simulink model "testMPC"  (R2019a)
settings: Solver=VariableStepAuto  StartTime=0.0  StopTime=10000  RelTol=1e-3
values from neighbouring files (symbols this model uses):
  Afault1_2 = [-0.0777422601611 0 0.00516641602336 0 0 0 0 0 0 1 0 0.364315718282 ... (121 elements, 11x11)]    [UpdatedWorkspace.mat]    (also in current.mat; current2.mat; finalWorkspace.mat; genTestingData.m = [-0.0777422601610909,0.364315718281914,0,-49.5311012194985,0)
  Bfault1_2 = [0 -0.116933195054 -1.86328082403 0 0 0 0 0 0 0 0 0 ... (44 elements, 11x4)]    [UpdatedWorkspace.mat]    (also in current.mat; current2.mat; finalWorkspace.mat; genTestingData.m = [0,0,0,0)
  C = [1 0 0 0 0 0 0 0 0 0 0 ... (first row only)    [chanceConstraintProgramming4.m]    (also in current.mat = [1 0 0 0 0 0 0 0 0 0 0 0 ... (44 elements, 4x11)]; current2.mat = [1 0 0 0 0 0 0 0 0 0 0 0 ... (44 elements, 4x11)])
undefined symbols (not defined in the file or in its folder): testA, testB
libraries: mpclib x1
settings Model: Creator=mschr  LastModifiedBy=mschr

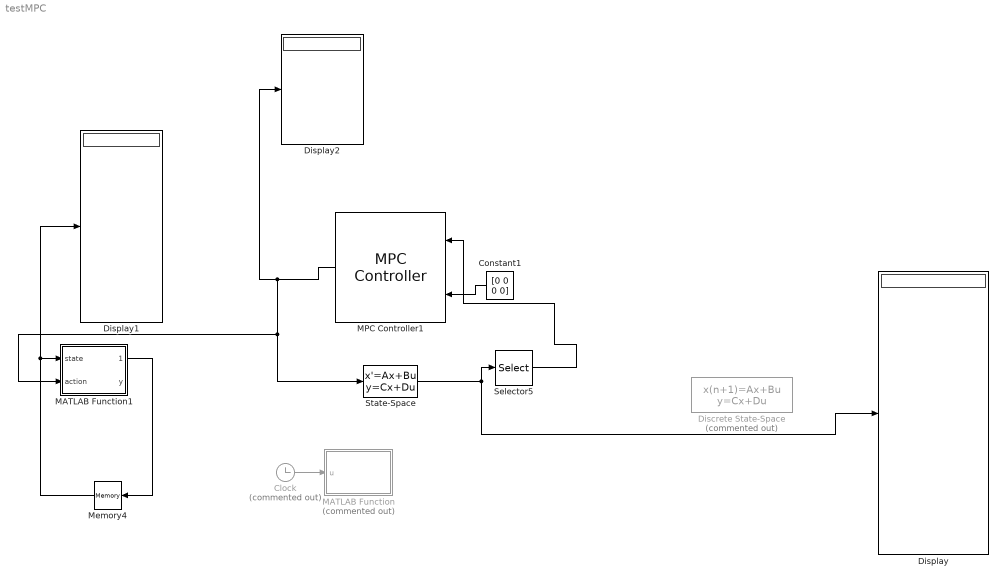
== system testMPC ==
  Clock : Clock  Commented=on
  Constant1 : Constant  Value=[0 0 0 0]
  Discrete State-Space : DiscreteStateSpace  Commented=on  A=testA  B=testB  C=C  D=zeros(4,4)  InitialCondition=[160 0 0 0 0 0 0 0 0 0 0]  SampleTime=-1
  Display : Display
  Display1 : Display
  Display2 : Display
  MATLAB Function : MATLAB Function  Commented=on  TreatAsAtomicUnit=on
  MATLAB Function1 : MATLAB Function  TreatAsAtomicUnit=on
  MPC Controller1 : mpclib/MPC Controller  SCDEnableBlockLinearizationSpecification=on  is_multiple=0  enable_value=0  return_u0=off  updateMPCinCallerWorkspace=on  md_inport=off  mv_inport=off  uref_inport=off  return_cost=off  return_mvseq=off  return_qpstatus=off  return_xseq=off  return_state=off  return_ovseq=off  state_inport=off  umin_inport=off  umax_inport=off  ymin_inport=off  ymax_inport=off  cc_inport=off  ywt_inport=off  uwt_inport=off  duwt_inport=off  rhoeps_inport=off  pm_inport=off  MaximumP=10  HorizonChoice=FixedHorizon  n_ts=0.05  n_p=70  n_mv=4  n_md=0  n_ud=0  n_mo=4  n_uo=0  BlockDataType=double  SampleTimeInherited=off  switch_inport=off
      settings: SourceProductName=MATLAB Runtime - Model Predictive Control Toolbox Addin  SourceProductBaseCode=Missing
  Memory4 : Memory  InitialCondition=[1 0 0 0 0 0 0 0 0 0 -50]  InheritSampleTime=on  LinearizeAsDelay=on
  Selector5 : Selector  InputPortWidth=11  IndexOptions=Index vector (dialog)  Indices=[1 8 9 11]  OutputSizes=1
  State-Space : StateSpace  A=Afault1_2  B=Bfault1_2  C=eye(11)  D=zeros(11,4)  InitialCondition=[1 0 0 0 0 0 0 10 5 0 -1]
  wires:
  Constant1/1 -> MPC Controller1/2
  MPC Controller1/1 -> MATLAB Function1/2(action), State-Space/1, Display2/1
  State-Space/1 -> Selector5/1, Display/1
  Clock/1 -> MATLAB Function/1(u)
  Selector5/1 -> MPC Controller1/1
  MATLAB Function1/1(nextState) -> Memory4/1
  Memory4/1 -> Display1/1, MATLAB Function1/1(state)

== matlab function testMPC/MATLAB Function1 ==
  data: nextState output; state input; y output; action input
function [nextState,y] = fcn2(state, action)
Anominal=[-0.0220400000000000,0.00142200000000000,0,-32.1700000000000,0,0,0,0,0,0,0;
    -0.0575900000000000,-0.394300000000000,871,0,0,0,0,0,0,0,0;
    -9.50000000000000e-05,-0.00179300000000000,-0.546800000000000,0,0,0,0,0,0,0,0;
    0,0,1,0,0,0,0,0,0,0,0;
    0,0,0,0,-0.0639900000000000,0,-1,0.0369100000000000,0,0,0;
    0,0,0,0,-2.11100000000000,-0.504800000000000,0.193000000000000,0,0,0,0;
    0,0,0,0,0.773200000000000,0.0108700000000000,-0.179400000000000,0,0,0,0;
    0,0,0,0,0,1,0,0,0,0,0;
    0,0,0,0,0,0,1,0,0,0,0;
    1,0,0,0,0,0,0,0,0,0,0;
    0,1,0,0,0,0,0,0,0,0,0];
Bnominal=[0,1.91000000000000e-05,0,0;
    -18.5800000000000,0,0,0;
    -1.20000000000000,0,0,0;
    0,0,0,0;
    0,0,0,0.00839000000000000;
    0,0,0.184800000000000,0.105600000000000;
    0,0,-0.00869900000000000,-0.459100000000000;
    0,0,0,0;
    0,0,0,0;
    0,0,0,0;
    0,0,0,0];

Afault2=[-0.0220400000000000,0.00142200000000000,0,-32.1700000000000,0,0,0,0,0,0,0;
    -0.0575900000000000,-0.394300000000000,871,0,0,0,0,0,0,0,0;
    -9.50000000000000e-05,-0.00179300000000000,-0.546800000000000,0,0,0,0,0,0,0,0;
    0,0,1,0,0,0,0,0,0,0,0;
    0,0,0,0,0,-0.00110800000000000,-1,0.0369100000000000,0,0,0;
    0,0,0,0,-1.23500000000000,-0.481800000000000,0.0891100000000000,0,0,0,0;
    0,0,0,0,0,-0.0519300000000000,0,0,0,0,0;
    0,0,0,0,0,1,0,0,0,0,0;
    0,0,0,0,0,0,1,0,0,0,0;
    1,0,0,0,0,0,0,0,0,0,0;
    0,1,0,0,0,0,0,0,0,0,0];
Bfault2=[0,1.91000000000000e-05,0,0;
    -18.5800000000000,0,0,0;
    -1.20000000000000,0,0,0;
    0,0,0,0;
    0,0,0,0;
    0,0,0.187900000000000,0;
    0,0,0,0;
    0,0,0,0;
    0,0,0,0;
    0,0,0,0;
    0,0,0,0];

Afault1_2=[-0.0777422601610909,0.364315718281914,0,-49.5311012194985,0,0,0,0,0,0,0;
    0,-2.11693319505418,-8.082029025490,0,0,0,0,0,0,0,0;
    0.00516641602336364,-3.5543885272319,-2.926680000000,-2.37481704217243,0,0,0,0,0,0,0;
    0,0,1,0,0,0,0,0,0,0,0;
    0,0,0,0,-1.73568157299046,-0.00695689900121296,-246.715568807515,49.5311012194985,0,0,0;
    0,0,32.90144280000,31.3713331270978,-0.0210854784922154,-0.00633571574984461,0.00174212652554297,0,0,0,0;
    0,0,0,13.2100000000000,0.0233794202315124,-4.26083552968259e-05,-0.00576851579403181,0,0,0,0;
    0,0,0,0,0,1,0.0479459770467924,0,0,0,0;
    0,0,0,0,0,0,1,0,0,0,0;
    1,0,0,0,0,0,0,0,0,0,0;
    0,1,0,0,0,0,0,0,0,0,0]
Bfault1_2=[0,0,0,0;
    -.11693319505418,0,0,0;
    -1.863280824027,0,0,0;
    0,0,0,0;
    0,0,0,-0.00412083182815909;
    0,0,0.00602442242634726,0.00602442242634726;
    0,0,0,-0.0221156677865658;
    0,0,0,0;0,0,0,0;0,0,0,0;0,0,0,0]
 
Afault1=[-0.00470000000000000,-0.0107700000000000,0,-623300,0,0,0,0,0,0,0;
     -0.310000000000000,-0.253000000000000,16780000,-28300,0,0,0,0,0,0,0;
     0,0,-157900,264.600000000000,0,0,0,0,0,0,0;
     0,0,1,0,0,0,0,0,0,0,0;
     0,0,0,0,-0.0470000000000000,0,-16890000,620000,0,0,0;
     0,0,463000,-7797,-0.00160000000000000,-0.201300000000000,0.105500000000000,0,0,0,0;
     0,0,0,171900,0.000570000000000000,-0.00650000000000000,-157900,5833,0,0,0;
     0,0,0,0,0,1,0.0454100000000000,0,0,0,0;
     0,0,0,0,0,0,1,0,0,0,0;
     1,0,0,0,0,0,0,0,0,0,0;
     0,871,0,0,0,0,0,0,0,0,0];
 Bfault1=[0,0,0,0;
     13.3300000000000,0,0,0;
     -0.914700000000000,0,0,0;
     0,0,0,0;
     0,0,0,5.37700000000000;
     0,0,0.0670800000000000,0.0762900000000000;
     0,0,13.3200000000000,-0.289500000000000;
     0,0,0,0;
     0,0,0,0;
     0,0,0,0;
     0,0,0,0];
% C=[1,0,0,0,0,0,0,0,0,0,0;
%     0,0,0,1,0,0,0,0,0,0,0;
%     0,0,0,0,0,0,0,1,0,0,0;
%     0,0,0,0,0,0,0,0,1,0,0;
%     0,0,0,0,0,0,0,0,0,1,0;
%     0,0,0,0,0,0,0,0,0,0,1]
 %y=zeros(6,1);
deltaS=zeros(11,1)
Anominal*state
state
     deltaS=Afault1_2*state*.05+Bfault1_2*action*.05;
     nextState=deltaS+state
    y=nextState


end

== matlab function testMPC/MATLAB Function ==
  data: u input
function fcn(u)
coder.extrinsic('mat2str')
coder.extrinsic('set_param')
Afault1_2=[-0.0777422601610909,0.364315718281914,0,-49.5311012194985,0,0,0,0,0,0,0;0,-2.11693319505418,-8.08202902549000,0,0,0,0,0,0,0,0;0.00516641602336364,-3.55438852723190,-2.92668000000000,-2.37481704217243,0,0,0,0,0,0,0;0,0,1,0,0,0,0,0,0,0,0;0,0,0,0,-1.73568157299046,-0.00695689900121296,-246.715568807515,49.5311012194985,0,0,0;0,0,32.9014428000000,31.3713331270978,-0.0210854784922154,-0.00633571574984461,0.00174212652554297,0,0,0,0;0,0,0,13.2100000000000,0.0233794202315124,-4.26083552968259e-05,-0.00576851579403181,0,0,0,0;0,0,0,0,0,1,0.0479459770467924,0,0,0,0;0,0,0,0,0,0,1,0,0,0,0;1,0,0,0,0,0,0,0,0,0,0;0,1,0,0,0,0,0,0,0,0,0]
Bfault1_2=[0,1.91000000000000e-05,0,0;-0.116933195054180,0,0,0;-1.86328082402700,0,0,0;0,0,0,0;0,0,0,-0.00412083182815909;0,1.91000000000000e-08,0.00602442242634726,0.00602442242634726;0,0,0,-0.0221156677865658;0,0,0,0;0,0,0,0;0,0,0,0;0,0,0,0]
Anominal=[-0.0220400000000000,0.00142200000000000,0,-32.1700000000000,0,0,0,0,0,0,0;
    -0.0575900000000000,-0.394300000000000,871,0,0,0,0,0,0,0,0;
    -9.50000000000000e-05,-0.00179300000000000,-0.546800000000000,0,0,0,0,0,0,0,0;
    0,0,1,0,0,0,0,0,0,0,0;
    0,0,0,0,-0.0639900000000000,0,-1,0.0369100000000000,0,0,0;
    0,0,0,0,-2.11100000000000,-0.504800000000000,0.193000000000000,0,0,0,0;
    0,0,0,0,0.773200000000000,0.0108700000000000,-0.179400000000000,0,0,0,0;
    0,0,0,0,0,1,0,0,0,0,0;
    0,0,0,0,0,0,1,0,0,0,0;
    1,0,0,0,0,0,0,0,0,0,0;
    0,1,0,0,0,0,0,0,0,0,0];
Bnominal=[0,1.91000000000000e-05,0,0;
    -18.5800000000000,0,0,0;
    -1.20000000000000,0,0,0;
    0,0,0,0;
    0,0,0,0.00839000000000000;
    0,0,0.184800000000000,0.105600000000000;
    0,0,-0.00869900000000000,-0.459100000000000;
    0,0,0,0;
    0,0,0,0;
    0,0,0,0;
    0,0,0,0];

if u>100
    set_param('testMPC/At','A',mat2str(Afault1_2),'B',mat2str(Bfault1_2))
else
    set_param('testMPC/At','A',mat2str(Anominal),'B',mat2str(Bnominal))
end

y = u;
